simulink library "Lib_Cntrl_SetPoint_TMATS"  (R2015a)
settings: Solver=ode45  StartTime=0.0  StopTime=10.0  RelTol=1e-3
Description:
  | Thomas Modules
settings Model: Creator=jwchapm2  LastModifiedBy=jwchapm2
settings OptimizationCC: ExpressionDepthLimit=2147483647
settings DebuggingCC: UnderspecifiedInitializationDetection=Classic  MergeDetectMultiDrivingBlocksExec=none  SolverPrmCheckMsg=warning  StateNameClashWarn=warning

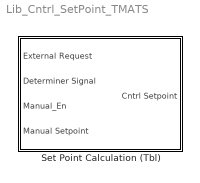
== system Lib_Cntrl_SetPoint_TMATS ==
  Set Point Calculation (Tbl) : Subsystem  mask(T-MATS: Set Point Calculation (Tbl)){ERVec_M=[1 2], DSVec_M=[1 2 3], SPArray_M=[1 1 1;2 2 2]}
      mask prompts: ERVec_M "ERVec_M - External request vector (1xm)"; DSVec_M "DSVec_M - Determiner signal vector (1xn)"; SPArray_M "SPArray_M - Set point array (SP = f(ER,DS)) (mxn)"
      mask help: This block contains a set point table look up based on an external request and a manual override.
      mask Help: web(which('Control_TMATS_SPCalc.html'),'-helpbrowser')

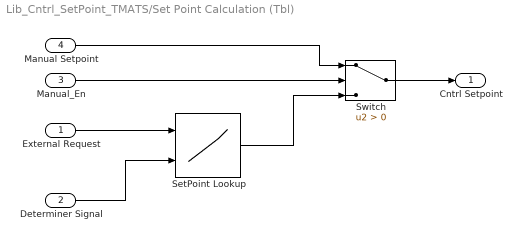
== system Lib_Cntrl_SetPoint_TMATS/Set Point Calculation (Tbl) ==
  External Request : Inport
  Determiner Signal : Inport  Port=2
  Manual_En : Inport  Port=3
  Manual Setpoint : Inport  Port=4
  SetPoint Lookup : Lookup_n-D  BreakpointsForDimension1=ERVec_M  BreakpointsForDimension2=DSVec_M  Table=SPArray_M  InternalRulePriority=Speed  RndMeth=Simplest  InputSameDT=on
  Switch : Switch  Criteria=u2 > Threshold
  Cntrl Setpoint : Outport
  wires:
  Determiner Signal/1 -> SetPoint Lookup/2
  External Request/1 -> SetPoint Lookup/1
  SetPoint Lookup/1 -> Switch/3
  Switch/1 -> Cntrl Setpoint/1
  Manual Setpoint/1 -> Switch/1
  Manual_En/1 -> Switch/2
